simulink model "Selector_TestGen8"  (R2017b)
settings: Solver=FixedStepDiscrete  StartTime=0.0  StopTime=10.0  RelTol=1e-3
undefined symbols (not defined in the file): Block_TestLib, trigger
settings Model: Creator=ktrinh  LastModifiedBy=ktrinh
settings DebuggingCC: ParameterOverflowMsg=none

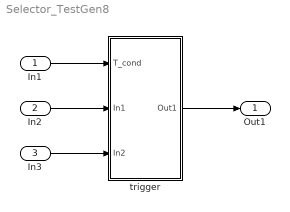
== system Selector_TestGen8 ==
  In1 : Inport
  In2 : Inport  Port=2
  In3 : Inport  Port=3
  trigger : Subsystem  AncestorBlock=Block_TestLib/trigger
  Out1 : Outport
  wires:
  In1/1 -> trigger/1(T_cond)
  In2/1 -> trigger/2(In1)
  In3/1 -> trigger/3(In2)
  trigger/1(Out1) -> Out1/1

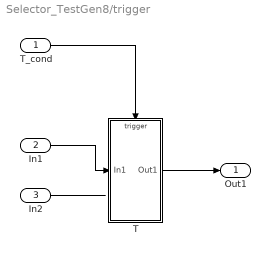
== system Selector_TestGen8/trigger ==
  T_cond : Inport  OutDataTypeStr=boolean
  In1 : Inport  Port=2
  In2 : Inport  Port=3
  T : Subsystem  TreatAsAtomicUnit=on
  Out1 : Outport
  wires:
  T_cond/1 -> T/Trigger
  In1/1 -> T/1(In1)
  In2/1 -> ?
  T/1(Out1) -> Out1/1

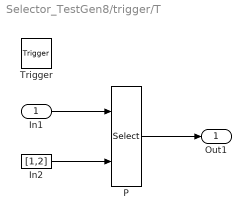
== system Selector_TestGen8/trigger/T ==
  In1 : Inport  OutDataTypeStr=int8  PortDimensions=[2 2]
  Trigger : TriggerPort  VariantControl=Variant
  In2 : Constant  Value=[1,2]
  P : Selector  NumberOfDimensions=2  InputPortWidth=3  IndexOptions=Index vector (port),Starting index (dialog)  Indices=[],1  OutputSizes=,2
  Out1 : Outport
  wires:
  In1/1 -> P/1
  In2/1 -> P/2
  P/1 -> Out1/1
